simulink model "balanceOfPlant"  (R2023a)
settings: Solver=FixedStepAuto  StartTime=0.0  StopTime=10.0  FixedStep=0.001  RelTol=1e-3
libraries: slpidlib x1
settings Model: Creator=thomas-guilbaud  LastModifiedBy=thomas-guilbaud
settings SolverCC: ConcurrentTasks=on  PositivePriorityOrder=on
settings OptimizationCC: BlockReduction=off  OptimizeBlockIOStorage=off
settings DebuggingCC: AlgebraicLoopMsg=none  TasksWithSamePriorityMsg=none  DebugExecutionForFMUViaOutOfProcess=on
settings HardwareCC: TargetBitPerLong=64  TargetBitPerPointer=64  TargetBitPerSizeT=64  TargetBitPerPtrDiffT=64  TargetLongLongMode=on  TargetIntDivRoundTo=Zero  TargetEndianess=LittleEndian  TargetWordSize=64  TargetHWDeviceType=MATLAB Host  ProdEqTarget=off
settings RTWCC: Toolchain=Simulink Real-Time Toolchain  BuildConfiguration=Faster Runs
settings GRTTargetCC: CombineOutputUpdateFcns=off

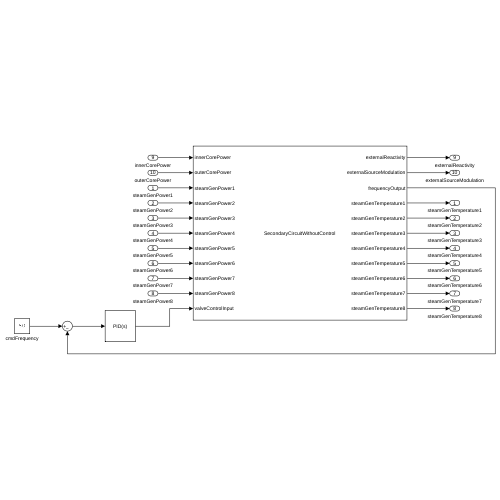
[thumbnail: Simulink's stored preview of the top-level diagram]
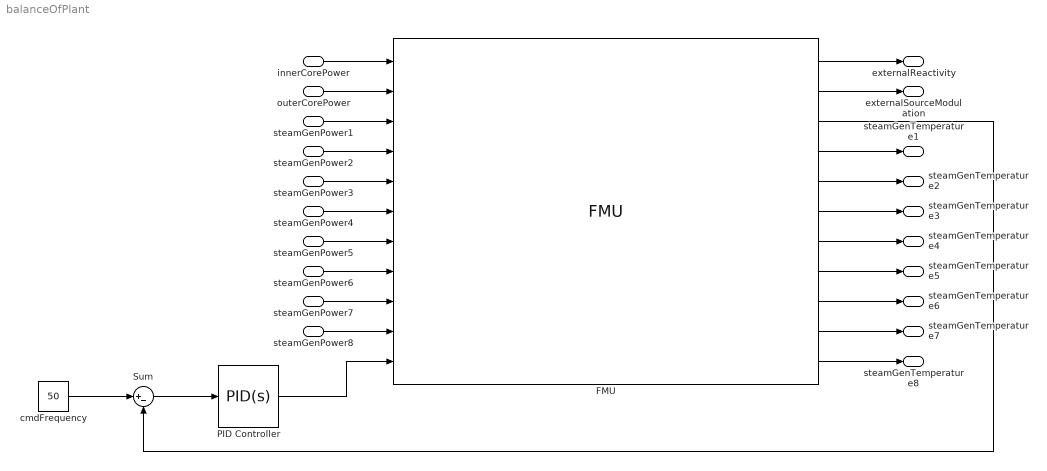
== system balanceOfPlant ==
  steamGenPower1 : Inport
  steamGenPower2 : Inport  Port=2
  steamGenPower3 : Inport  Port=3
  steamGenPower4 : Inport  Port=4
  steamGenPower5 : Inport  Port=5
  steamGenPower6 : Inport  Port=6
  steamGenPower7 : Inport  Port=7
  steamGenPower8 : Inport  Port=8
  innerCorePower : Inport  Port=9
  outerCorePower : Inport  Port=10
  FMU : FMU  FMUName=SecondaryCircuitWithoutControl.fmu  FMUMode=CoSimulation  HP=struct('Kt',0.0055,'eta_iso_nom',0.7,'eta_mech',0.7)  Ku=0.25  KuExtSrc=1e-09  KuReact=1e-12  LP1=struct('Kt',0.00929,'eta_iso_nom',0.7,'eta_mech',0.7)  LP2=struct('Kt',0.00929,'eta_iso_nom',0.7,'eta_mech',0.7)  SG1=struct('Cfnom',0.0,'Kfc',1.0,'Kfnom',0.0,'dpnom',0.0,'e',0.0,'heatTransfer',struct('kc',1.0),'hstartin',1541000.0,'hstartout',1732000.0,'rhonom',0.0,'wnf',0.02,'FluidPhaseStart',int32(1))  SG2=struct('Cfnom',0.0,'Kfc',1.0,'Kfnom',0.0,'dpnom',0.0,'e',0.0,'heatTransfer',struct('kc',1.0),'hstartin',1732000.0,'hstartout',1889000.0,'rhonom',0.0,'wnf',0.02,'FluidPhaseStart',int32(1))  SG3=struct('Cfnom',0.0,'Kfc',1.0,'Kfnom',0.0,'dpnom',0.0,'e',0.0,'heatTransfer',struct('kc',1.0),'hstartin',1889000.0,'hstartout',1978000.0,'rhonom',0.0,'wnf',0.02,'FluidPhaseStart',int32(3))  SG4=struct('Cfnom',0.0,'Kfc',1.0,'Kfnom',0.0,'dpnom',0.0,'e',0.0,'heatTransfer',struct('kc',1.0),'hstartin',1978000.0,'hstartout',2106000.0,'rhonom',0.0,'wnf',0.02,'FluidPhaseStart',int32(3))  SG5=struct('Cfnom',0.0,'Kfc',1.0,'Kfnom',0.0,'dpnom',0.0,'e',0.0,'heatTransfer',struct('kc',1.0),'hstartin',2106000.0,'hstartout',2361000.0,'rhonom',0.0,'wnf',0.02,'FluidPhaseStart',int32(3))  SG6=struct('Cfnom',0.0,'Kfc',1.0,'Kfnom',0.0,'dpnom',0.0,'e',0.0,'heatTransfer',struct('kc',1.0),'hstartin',2361000.0,'hstartout',2689000.0,'rhonom',0.0,'wnf',0.02,'FluidPhaseStart',int32(3))  SG7=struct('Cfnom',0.0,'Kfc',1.0,'Kfnom',0.0,'dpnom',0.0,'e',0.0,'heatTransfer',struct('kc',1.0),'hstartin',2689000.0,'hstartout',2985000.0,'rhonom',0.0,'wnf',0.02,'FluidPhaseStart',int32(2))  SG8=struct('Cfnom',0.0,'Kfc',1.0,'Kfnom',0.0,'dpnom',0.0,'e',0.0,'heatTransfer',struct('kc',1.0),'hstartin',2985000.0,'hstartout',3083000.0,'rhonom',0.0,'wnf',0.02,'FluidPhaseStart',int32(2))  Tu=0.2  TuExtSrc=2.5  TuReact=2.5  add=struct('k1',1.0,'k2',1.0)  add3=struct('k1',1.0,'k2',1.0,'k3',1.0)  addPowers=struct('k1',1.0,'k2',1.0)  const=struct('k',120000000.0)  corePowerMeasure=struct('k',14276.2644)  defaultValve=struct('k',0.285)  gain=struct('k',2.5)  generator=struct('D',0.01,'Pnom',125000000.0,'Ta',10.0,'Tf',1.0,'eta',1.0,'system',struct('T_amb',293.15,'T_wb',288.15,'fnom',50.0,'p_amb',101325.0,'initOpt',int32(2)),'thetastart',0.0)  greaterThreshold=struct('threshold',0.5)  greaterThreshold1=struct('threshold',0.5)  inertia=struct('J',1000.0)  innerTubeDiameter=0.01905  interP=6000000.0  limiter=struct('uMax',1.0,'uMin',0.01)  load=struct('Pnom',125000000.0)  maxP=18800000.0  minP=8000.0  outerTubeDiameter=0.0254  pidExternalSource=struct('D',struct('y_start',0.0),'FFzero',struct('k',0.0),'Nd',10.0,'Ni',0.9,'P',struct('k',1.0),'addD',struct('k2',-1.0),'addFF',struct('k1',1.0),'addI',struct('k1',1.0,'k2',-1.0,'k3',1.0),'addP',struct('k2',-1.0),'addPID',struct('k1',1.0,'k2',1.0,'k3',1.0),'addSat',struct('k1',1.0,'k2',-1.0),'kFF',1.0,'limiter',struct('uMax',1.2,'uMin',0.0),'wd',0.0,'wp',1.0,'xd_start',0.0,'xi_start',0.0)  pidReactivity=struct('D',struct('y_start',0.0),'FFzero',struct('k',0.0),'Nd',10.0,'Ni',0.9,'P',struct('k',1.0),'addD',struct('k2',-1.0),'addFF',struct('k1',1.0),'addI',struct('k1',1.0,'k2',-1.0,'k3',1.0),'addP',struct('k2',-1.0),'addPID',struct('k1',1.0,'k2',1.0,'k3',1.0),'addSat',struct('k1',1.0,'k2',-1.0),'kFF',1.0,'limiter',struct('uMax',0.0025,'uMin',-0.0025),'wd',0.0,'wp',1.0,'xd_start',0.0,'xi_start',0.0)  pinPitch=0.0450566  rampLoad=struct('duration',10.0,'height',-20000000.0,'offset',0.0,'startTime',1000000000000000.0)  rampLoad2=struct('duration',10.0,'height',20000000.0,'offset',0.0,'startTime',1000000000000000.0)  signalProcess1=struct('maxValue',30000000.0,'minValue',0.0)  signalProcess2=struct('maxValue',30000000.0,'minValue',0.0)  signalProcess3=struct('maxValue',30000000.0,'minValue',0.0)  signalProcess4=struct('maxValue',30000000.0,'minValue',0.0)  signalProcess5=struct('maxValue',30000000.0,'minValue',0.0)  signalProcess6=struct('maxValue',30000000.0,'minValue',0.0)  signalProcess7=struct('maxValue',30000000.0,'minValue',0.0)  signalProcess8=struct('maxValue',30000000.0,'minValue',0.0)  sinkPressure=struct('T',314.0,'h',100000.0)  sourcePressure=struct('T',608.15,'h',100000.0)  steamGenBayonnet=struct('Cfnom',0.0,'Kfc',1.0,'Kfnom',0.0,'dpnom',0.0,'e',0.0,'heatTransfer',struct('kc',1.0),'hstartin',1000000.0,'hstartout',1540000.0,'omega',0.0,'rhonom',0.0,'wnf',0.02,'FluidPhaseStart',int32(3),'avoidInletEnthalpyDerivative',boolean(true))  stepActivateExtReactivity=struct('height',-1.0,'offset',1.0,'startTime',1000000000000000.0)  stepActivateExtSource=struct('height',-1.0,'offset',1.0,'startTime',1000000000000000.0)  system=struct('T_amb',293.15,'T_wb',288.15,'fnom',50.0,'p_amb',101325.0,'initOpt',int32(2))  valveLiqChoked=struct('Av',0.1,'Cv',0.0,'Flnom',0.9,'Kv',0.0,'b',0.01,'dpnom',100.0,'rhonom',1000.0,'theta_fix',1.0,'thetanom',1.0)  valveVapAdmissionTurb=struct('Av',0.2,'Cv',0.0,'Fxt_full',0.5,'Kv',0.0,'b',0.01,'dpnom',999.9999999999999,'rhonom',80.0,'theta_fix',1.0,'thetanom',1.0)  valveVapBypass=struct('Av',0.5,'Cv',0.0,'Fxt_full',0.5,'Kv',0.0,'b',0.01,'dpnom',10000.0,'rhonom',80.0,'theta_fix',0.0,'thetanom',1.0)  volumetricArea=56.69862  wnm=1.0  wnom=192.7  nSGparallel=int32(8)  flowJoin=struct('checkFlowDirection',boolean(false))  flowJoinTurbLP=struct('checkFlowDirection',boolean(false))  flowSplitBypass=struct('checkFlowDirection',boolean(false))  flowSplitTurbLP=struct('checkFlowDirection',boolean(false))  mask(SecondaryCircuitWithoutControl [Co-Simulation, v2.0]){}
      mask Display:
      | disp('SecondaryCircuitWithoutControl');
      | port_label('output',1,'externalReactivity');
      | port_label('output',2,'externalSourceModulation');
      | port_label('output',3,'frequencyOutput');
      | port_label('output',4,'steamGenTemperature1');
      | port_label('output',5,'steamGenTemperature2');
      | port_label('output',6,'steamGenTemperature3');
      | port_label('output',7,'steamGenTemperature4');
      | port_label('output',8,'steamGenTemperature5');
      | port_label('output',9,'steamGenTemperature6');
      | port_label('output',10,'steamGenTemperature7');
      | port_label('output',11,'steamGenTemperature8');
      | port_label('input',1,'innerCorePower');
      | port_label('input',2,'outerCorePower');
      | port_label('input',3,'steamGenPower1');
      | port_label('input',4,'steamGenPower2');
      | port_label('input',5,'steamGenPower3');
      | port_label('input',6,'steamGenPower4');
      | port_label('input',7,'steamGenPower5');
      | port_label('input',8,'steamGenPower6');
      | port_label('input',9,'steamGenPower7');
      | port_label('input',10,'steamGenPower8');
      | port_label('input',11,'valveControlInput');
  PID Controller : slpidlib/PID Controller  Controller=PID  Form=Ideal  TimeDomain=Continuous-time  UseExternalTs=off  SampleTime=-1  IntegratorMethod=Forward Euler  FilterMethod=Forward Euler  ControllerParametersSource=internal  P=0.05  I=1/(0.2*0.5)  UseKiTs=off  D=0.33*0.2  N=10  UseFilter=on  TunerSelectOption=Transfer Function Based (PID Tuner App)  ZeroCross=off  InitialConditionSource=internal  InitialConditionForIntegrator=0  InitialConditionForFilter=0  DifferentiatorICPrevScaledInput=0  ExternalReset=none  TrackingMode=off  Kt=1  LimitOutput=off  SatLimitsSource=internal  UpperSaturationLimit=1  LowerSaturationLimit=0  LinearizeAsGain=on  AntiWindupMode=none  Kb=1  LimitIntegrator=off  UpperIntegratorSaturationLimit=inf  LowerIntegratorSaturationLimit=-inf  POutMin=[]  POutMax=[]  IOutMin=[]  IOutMax=[]  DOutMin=[]  DOutMax=[]  NOutMin=[]  NOutMax=[]  SumOutMin=[]  SumOutMax=[]  SaturationOutMin=[]  SaturationOutMax=[]  PParamMin=[]  PParamMax=[]  IParamMin=[]  IParamMax=[]  DParamMin=[]  DParamMax=[]  NParamMin=[]  NParamMax=[]  KbParamMin=[]  KbParamMax=[]  KtParamMin=[]  KtParamMax=[]  KbOutMin=[]  KbOutMax=[]  KtOutMin=[]  KtOutMax=[]  IntegratorOutMin=[]  IntegratorOutMax=[]  FilterOutMin=[]  FilterOutMax=[]  SumI1OutMin=[]  SumI1OutMax=[]  SumI2OutMin=[]  SumI2OutMax=[]  SumI3OutMin=[]  SumI3OutMax=[]  SumI4OutMin=[]  SumI4OutMax=[]  SumDOutMin=[]  SumDOutMax=[]  DifferentiatorOutMin=[]  DifferentiatorOutMax=[]  FilterDiffOutCoefMin=[]  FilterDiffOutCoefMax=[]  ReciprocalOutMin=[]  ReciprocalOutMax=[]  SumDenOutMin=[]  SumDenOutMax=[]  SumNumOutMin=[]  SumNumOutMax=[]  DivideOutMin=[]  DivideOutMax=[]  UdiffTsProdOutMin=[]  UdiffTsProdOutMax=[]  NTsProdOutMin=[]  NTsProdOutMax=[]  UintegralTsProdOutMin=[]  UintegralTsProdOutMax=[]  UngainTsProdOutMin=[]  UngainTsProdOutMax=[]  ClampingZeroOutDataTypeStr=Inherit: Inherit via back propagation  ClampingZeroOutMin=[]  ClampingZeroOutMax=[]  FilterDenConstantOutDataTypeStr=Inherit: Inherit via back propagation  FilterDenConstantOutMin=[]  FilterDenConstantOutMax=[]  PCopyOutDataTypeStr=Inherit: Inherit via back propagation  PCopyOutMin=[]  PCopyOutMax=[]  NCopyOutDataTypeStr=Inherit: Inherit via back propagation  NCopyOutMin=[]  NCopyOutMax=[]  IntegratorContinuousStateAttributes=''  IntegratorStateMustResolveToSignalObject=off  IntegratorRTWStateStorageClass=Auto  FilterContinuousStateAttributes=''  FilterStateMustResolveToSignalObject=off  FilterRTWStateStorageClass=Auto  ParallelPVariant=Passthrough  IdealPVariant=InternalParameters  IVariant=InternalParameters  DVariant=InternalParameters  IntegratorVariant=Continuous  SatVariant=Disabled  AWVariant=Passthrough  PCopyVariant=Disabled  TRVariant=Disabled  FdbkBlocksVariant=Forward  IdealPFdbkVariant=Disabled  SatFdbkVariant=Disabled  DerivativeFilterVariant=ContFilter  NVariant=InternalParameters  NCopyVariant=Disabled  FilterICVariant=InternalICsFilter  IntegratorICVariant=InternalICs  ExternalResetVariant=Disabled  TRSumVariant=Passthrough  SumFdbkVariant=Disabled  SumVariant=Sum_PID  TsampFilterVariant=InternalTs  TsampNgainVariant=Passthrough  TsampIntegralVariant=Disabled_SignalSpec  ExternalSaturationOutDataTypeStr=Inherit: Same as second input
  Sum : Sum  Inputs=|+-
  cmdFrequency : Constant  Value=50
  steamGenTemperature1 : Outport
  steamGenTemperature2 : Outport  Port=2
  steamGenTemperature3 : Outport  Port=3
  steamGenTemperature4 : Outport  Port=4
  steamGenTemperature5 : Outport  Port=5
  steamGenTemperature6 : Outport  Port=6
  steamGenTemperature7 : Outport  Port=7
  steamGenTemperature8 : Outport  Port=8
  externalReactivity : Outport  Port=9
  externalSourceModulation : Outport  Port=10
  wires:
  FMU/3 -> Sum/2
  Sum/1 -> PID Controller/1
  cmdFrequency/1 -> Sum/1
  PID Controller/1 -> FMU/11
  steamGenPower1/1 -> FMU/3
  steamGenPower2/1 -> FMU/4
  steamGenPower3/1 -> FMU/5
  steamGenPower4/1 -> FMU/6
  steamGenPower5/1 -> FMU/7
  steamGenPower6/1 -> FMU/8
  steamGenPower7/1 -> FMU/9
  steamGenPower8/1 -> FMU/10
  FMU/4 -> steamGenTemperature1/1
  FMU/5 -> steamGenTemperature2/1
  FMU/6 -> steamGenTemperature3/1
  FMU/7 -> steamGenTemperature4/1
  FMU/8 -> steamGenTemperature5/1
  FMU/9 -> steamGenTemperature6/1
  FMU/10 -> steamGenTemperature7/1
  FMU/11 -> steamGenTemperature8/1
  FMU/1 -> externalReactivity/1
  FMU/2 -> externalSourceModulation/1
  innerCorePower/1 -> FMU/1
  outerCorePower/1 -> FMU/2
